simulink model "ANNModel"  (R2020a)
settings: Solver=VariableStepAuto  StartTime=0.0  StopTime=10.0  RelTol=1e-3
values from neighbouring files (symbols this model uses):
  dijastolniPritisak = str2num(get(handles.edit2,'string'))    [GUI.m]
  glukoza = str2num(get(handles.edit4,'string'))    [GUI.m]
  obimStruka = str2num(get(handles.edit1,'string'))    [GUI.m]
  sistolniPritisak = str2num(get(handles.edit3,'string'))    [GUI.m]
  trigliceridi = str2num(get(handles.edit5,'string'))    [GUI.m]
undefined symbols (not defined in the file or in its folder): hdlCartesian2PolarSetting
libraries: neural x255
(part 4 of 4)

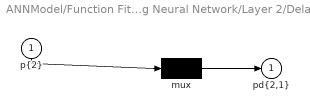
== system ANNModel/Function Fitting Neural Network/Layer 2/Delays 1 ==
  "p{2}" : Inport  PortDimensions=250
      mask Display: e = 0.06;c1 = [120 230 180]/255;c2 = ([120 230 180]+0)/(256+128);c3 = ([120 230 180]+128)/(256+128);patch([0 1 1 0],[0 0 1 1],c1);patch([0 1 1 1-e 1-e 0+e],[0 0 1 1-e 0+e 0+e],c2);patch([0 0 1 1-e 0+e 0+e],[0 1 1 1-e 1-e 0+e],c3);plot([0 1 1 0 0],[0 0 1 1 0]);
  mux : Mux  Inputs=1
      mask Display: e = 0.06;c1 = [120 150 230]/255;c2 = ([120 150 230]+0)/383;c3 = ([120 150 230]+128)/383;patch([0 1 1 0],[0 0 1 1],c1);patch([0 1 1 1-e 1-e 0+e],[0 0 1 1-e 0+e 0+e],c2);patch([0 0 1 1-e 0+e 0+e],[0 1 1 1-e 1-e 0+e],c3);plot([0 1 1 0 0],[0 0 1 1 0]);disp('Mux')
  "pd{2,1}" : Outport
      mask Display: e = 0.06;c1 = [120 230 180]/255;c2 = ([120 230 180]+0)/(256+128);c3 = ([120 230 180]+128)/(256+128);patch([0 1 1 0],[0 0 1 1],c1);patch([0 1 1 1-e 1-e 0+e],[0 0 1 1-e 0+e 0+e],c2);patch([0 0 1 1-e 0+e 0+e],[0 1 1 1-e 1-e 0+e],c3);plot([0 1 1 0 0],[0 0 1 1 0]);
  wires:
  "p{2}"/1 -> mux/1
  mux/1 -> "pd{2,1}"/1

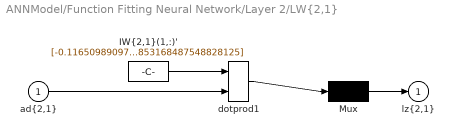
== system ANNModel/Function Fitting Neural Network/Layer 2/LW{2,1} ==
  "ad{2,1}" : Inport  PortDimensions=250
      mask Display: e = 0.06;c1 = [120 230 180]/255;c2 = ([120 230 180]+0)/(256+128);c3 = ([120 230 180]+128)/(256+128);patch([0 1 1 0],[0 0 1 1],c1);patch([0 1 1 1-e 1-e 0+e],[0 0 1 1-e 0+e 0+e],c2);patch([0 0 1 1-e 0+e 0+e],[0 1 1 1-e 1-e 0+e],c3);plot([0 1 1 0 0],[0 0 1 1 0]);
  "IW{2,1}(1,:)'" : Constant  Value=[-0.11650989097752244283423550541556323878467082977294921875;0.2440437508249433118390214758619549684226512908935546875;-0.053993313418870807207650130976617219857871532440185546875;-0.1312176258760666680558415464474819600582122802734375;0.038091512220755373296920964776290929876267910003662109375;0.00084023945522332973805113010001832662965171039104461669921875;-0.00128600288631221769397594556494368589483201503753662109375;-0.04565333781880025199040318284460227005183696746826171875;-0.1536371309185386169193776595420786179602146148681640625;0.1937446221878938723559571144505753181874752044677734375;0.1312113757065674068957861209128168411552906036376953125;0.10641759126912299360245839352501207031309604644775390625;0.0867090912659948254148645219174795784056186676025390625;0.075652792314880257240616856506676413118839263916015625;-0.0856915895263108684520858560063061304390430450439453125;0.0326858221364464129887750232228427194058895111083984375;0.17488457556046699270524413805105723440647125244140625;0.0254160445622617185701397346520025166682898998260498046875;-0.048367410191018145315666743044857867062091827392578125;-0.0023327369058948059683811226960870044422335922718048095703125;0.07658383350584518911574605226633138954639434814453125;-0.01313807539257783561781334213947047828696668148040771484375;0.0249156425127006926623085547589653288014233112335205078125;-0.0268333976484150422969765514835671638138592243194580078125;0.033353646039427871372584633036240120418369770050048828125;0.1550097168419988513665686014064704068005084991455078125;0.0197458018772514697081188472793655819259583950042724609375;0.012920988819453048390695215630330494605004787445068359375;0.05965495472012864730526615630878950469195842742919921875;-0.2025155294328965516204021923840628005564212799072265625;0.04167974585860954872540418136850348673760890960693359375;-0.0064437409467264471218950205866349278949201107025146484375;-0.10308807451588386516760920130764134228229522705078125;-0.0971787193204585453276678208567318506538867950439453125;0.005227177639702709592561813423117200727574527263641357421875;-0.039947943149199534318416482392422039993107318878173828125;0.13352178738392528334344433460501022636890411376953125;0.078439292975390484397024692952982150018215179443359375;-0.0281496176255796350107463155154619016684591770172119140625;0.11506888537159583318914002347810310311615467071533203125;-0.058144975675007370963243147343746386468410491943359375;-0.025820734449761385820298897897373535670340061187744140625;-0.06367816579818637301446671017401968128979206085205078125;-0.161432326305391005139000526469317264854907989501953125;-0.02223166266417241077046895725288777612149715423583984375;0.1660601092991398630704935612811823375523090362548828125;-0.048382574956638939311925895481181214563548564910888671875;0.01398818890455763401525768330202481593005359172821044921875;-0.1228716717678524361634373462948133237659931182861328125;-0.00867054350313501039082542121150254388339817523956298828125;-0.037203631600951116153996878210818977095186710357666015625;-0.0042475917452647928007625210966580198146402835845947265625;-0.0680539108959226368700257125965435989201068878173828125;-0.049276275434421916432636834315417218022048473358154296875;-0.1203392652723382083568282041596830822527408599853515625;0.01265474834338008169876133024445152841508388519287109375;-0.068284171343317101587899742298759520053863525390625;-0.1083372214501769625893956572326715104281902313232421875;-0.1193026703517045816749231335052172653377056121826171875;-0.0310748968969891715963260736543816165067255496978759765625;0.05871572949754337578109897322065080516040325164794921875;0.27242042871102878365263677551411092281341552734375;-0.0628473587753546336642784808645956218242645263671875;0.1753260138629249009767363531864248216152191162109375;0.0172062906358027949138556067509853164665400981903076171875;0.130283415814070158145199229693389497697353363037109375;-0.0037831506578785054593916381548979188664816319942474365234375 ...(+10847 chars)]
      mask Display: e = 0.06;c1 = [120 150 230]/255;c2 = ([120 150 230]+0)/383;c3 = ([120 150 230]+128)/383;patch([0 1 1 0],[0 0 1 1],c1);patch([0 1 1 1-e 1-e 0+e],[0 0 1 1-e 0+e 0+e],c2);patch([0 0 1 1-e 0+e 0+e],[0 1 1 1-e 1-e 0+e],c3);plot([0 1 1 0 0],[0 0 1 1 0]);disp('weights');
  Mux : Mux  Inputs=1
      mask Display: e = 0.06;c1 = [120 150 230]/255;c2 = ([120 150 230]+0)/383;c3 = ([120 150 230]+128)/383;patch([0 1 1 0],[0 0 1 1],c1);patch([0 1 1 1-e 1-e 0+e],[0 0 1 1-e 0+e 0+e],c2);patch([0 0 1 1-e 0+e 0+e],[0 1 1 1-e 1-e 0+e],c3);plot([0 1 1 0 0],[0 0 1 1 0]);disp('Mux');
  dotprod1 : neural/Weight Functions/dotprod
  "lz{2,1}" : Outport
      mask Display: e = 0.06;c1 = [120 230 180]/255;c2 = ([120 230 180]+0)/(256+128);c3 = ([120 230 180]+128)/(256+128);patch([0 1 1 0],[0 0 1 1],c1);patch([0 1 1 1-e 1-e 0+e],[0 0 1 1-e 0+e 0+e],c2);patch([0 0 1 1-e 0+e 0+e],[0 1 1 1-e 1-e 0+e],c3);plot([0 1 1 0 0],[0 0 1 1 0]);
  wires:
  "IW{2,1}(1,:)'"/1 -> dotprod1/1
  "ad{2,1}"/1 -> dotprod1/2
  dotprod1/1 -> Mux/1
  Mux/1 -> "lz{2,1}"/1
